simulink model "sg_pixel_blank_ML"  (Simulink 8.2)
settings: Solver=VariableStepDiscrete  StartTime=0.0  StopTime=Tsim  RelTol=1e-3
values from neighbouring files (symbols this model uses):
  ImgX = 640    [tb_pixel_blank_ML_xsvi_inout_only.m]    (also in tb_pixel_cnt.m = SizeI(2))
  ImgY = 480    [tb_pixel_blank_ML_xsvi_inout_only.m]    (also in tb_pixel_cnt.m = SizeI(1))
undefined symbols (not defined in the file or in its folder): gcbh, xlBlockLoadCallback, xlGetNormalizedPeriod
libraries: xbsIndex_r4 x73, dspsrcs4 x6
(part 1 of 2)
settings Model: Creator=sps  LastModifiedBy=tawassne
settings OptimizationCC: InitFltsAndDblsToZero=on
settings DebuggingCC: SaveWithParameterizedLinksMsg=none  SignalResolutionControl=TryResolveAllWithWarning  SolverPrmCheckMsg=none  MultiTaskDSMMsg=warning  MultiTaskCondExecSysMsg=none
settings RTWCC: IncludeERTFirstTime=on
settings GRTTargetCC: TargetFcnLib=ansi_tfl_tmw.mat

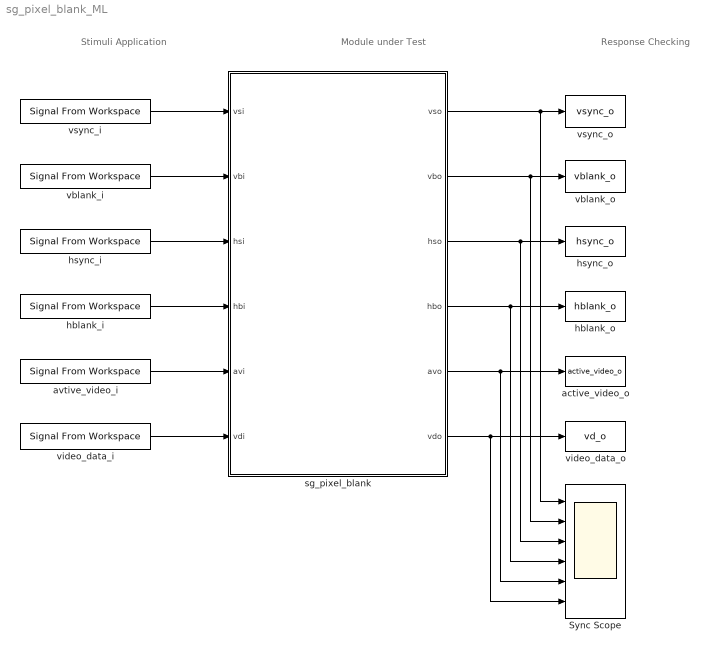
== system sg_pixel_blank_ML ==
  note: Stimuli Application
  note: Response Checking
  note: Module under Test
  Sync Scope : Scope  NumInputPorts=6
      settings: YMin=-5~-5~-5~-5~-5~-5  YMax=5~5~5~5~5~5
  active_video_o : ToWorkspace  VariableName=active_video_o  SampleTime=-1
      settings: MaxDataPoints=2*TFL
  avtive_video_i : dspsrcs4/Signal From Workspace  X=actvid_i  Ts=1  nsamps=1  OutputAfterFinalValue=Cyclic repetition  ignoreOrWarnInputAndFrameLengths=off
  hblank_i : dspsrcs4/Signal From Workspace  X=hblank_i  Ts=1  nsamps=1  OutputAfterFinalValue=Cyclic repetition  ignoreOrWarnInputAndFrameLengths=off
  hblank_o : ToWorkspace  VariableName=hblank_o  SampleTime=-1
      settings: MaxDataPoints=2*TFL
  hsync_i : dspsrcs4/Signal From Workspace  X=hsync_i  Ts=1  nsamps=1  OutputAfterFinalValue=Cyclic repetition  ignoreOrWarnInputAndFrameLengths=off
  hsync_o : ToWorkspace  VariableName=hsync_o  SampleTime=-1
      settings: MaxDataPoints=2*TFL
  sg_pixel_blank : Subsystem
  vblank_i : dspsrcs4/Signal From Workspace  X=vblank_i  Ts=1  nsamps=1  OutputAfterFinalValue=Cyclic repetition  ignoreOrWarnInputAndFrameLengths=off
  vblank_o : ToWorkspace  VariableName=vblank_o  SampleTime=-1
      settings: MaxDataPoints=2*TFL
  video_data_i : dspsrcs4/Signal From Workspace  X=vd_i  Ts=1  nsamps=1  OutputAfterFinalValue=Cyclic repetition  ignoreOrWarnInputAndFrameLengths=off
  video_data_o : ToWorkspace  VariableName=vd_o  SampleTime=-1
      settings: MaxDataPoints=2*TFL
  vsync_i : dspsrcs4/Signal From Workspace  X=vsync_i  Ts=1  nsamps=1  OutputAfterFinalValue=Cyclic repetition  ignoreOrWarnInputAndFrameLengths=off
  vsync_o : ToWorkspace  VariableName=vsync_o  SampleTime=-1
      settings: MaxDataPoints=2*TFL
  wires:
  vsync_i/1 -> sg_pixel_blank/1(vsi)
  vblank_i/1 -> sg_pixel_blank/2(vbi)
  hsync_i/1 -> sg_pixel_blank/3(hsi)
  hblank_i/1 -> sg_pixel_blank/4(hbi)
  avtive_video_i/1 -> sg_pixel_blank/5(avi)
  video_data_i/1 -> sg_pixel_blank/6(vdi)
  sg_pixel_blank/1(vso) -> vsync_o/1, Sync Scope/1
  sg_pixel_blank/2(vbo) -> vblank_o/1, Sync Scope/2
  sg_pixel_blank/3(hso) -> hsync_o/1, Sync Scope/3
  sg_pixel_blank/4(hbo) -> hblank_o/1, Sync Scope/4
  sg_pixel_blank/5(avo) -> active_video_o/1, Sync Scope/5
  sg_pixel_blank/6(vdo) -> video_data_o/1, Sync Scope/6

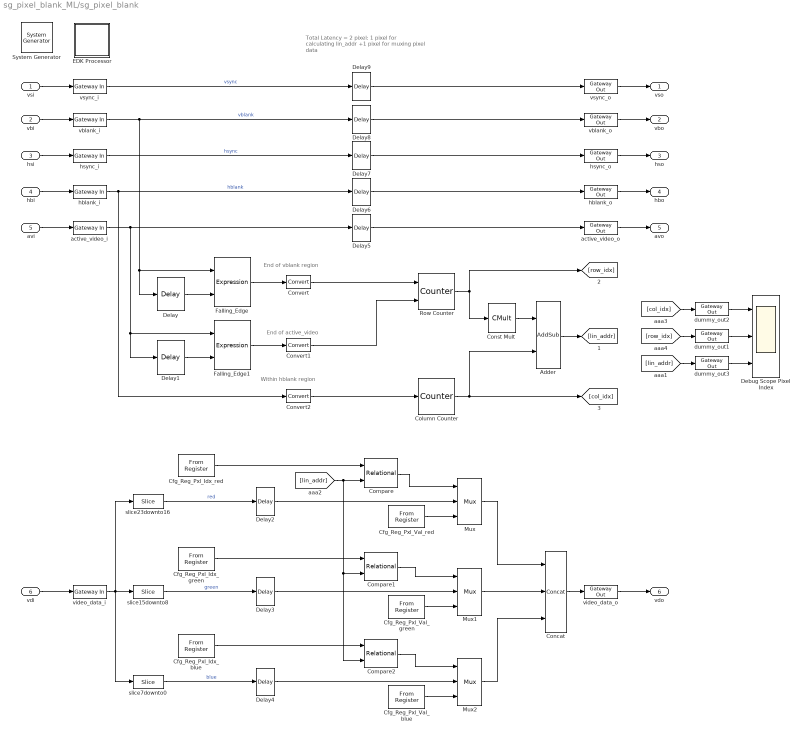
== system sg_pixel_blank_ML/sg_pixel_blank ==
  note: End of vblank region
  note: End of active_video
  note: Within hblank region
  note: Total Latency = 2 pixel:
      |     1 pixel for calculating lin_addr
      |   +1 pixel for muxing pixel data
  vsi : Inport
  vbi : Inport  Port=2
  hsi : Inport  Port=3
  hbi : Inport  Port=4
  avi : Inport  Port=5
  vdi : Inport  Port=6
  " System Generator" : xbsIndex_r4/ System Generator  Tag=genX  xilinxfamily=spartan6  part=xc6slx150t  speed=-3  package=fgg676  synthesis_tool=XST  clock_wrapper=Clock Enables  directory=./netlist  proj_type=Project Navigator  Synth_file=XST Defaults  Impl_file=ISE Defaults  testbench=off  simulink_period=1  sysclk_period=10  dcm_input_clock_period=10  incr_netlist=off  trim_vbits=Everywhere in SubSystem  dbl_ovrd=According to Block Masks  core_generation=According to Block Masks  run_coregen=off  deprecated_control=off  eval_field=0  block_type=sysgen
      settings: block_version=11.4
  Adder : xbsIndex_r4/AddSub  mode=Addition  use_carryin=off  use_carryout=off  en=off  latency=1  precision=Full  arith_type=Unsigned  n_bits=16  bin_pt=14  quantization=Truncate  overflow=Wrap  dbl_ovrd=off  use_behavioral_HDL=off  hw_selection=Fabric  pipelined=off  block_type=addsub
  Cfg_Reg_Pxl_Idx_blue : xbsIndex_r4/From Register  shared_memory_name='pixel_idx_blue'  init=70000  period=1  ownership=Locally owned and initialized  gui_display_data_type=Fixed-point  arith_type=Unsigned  n_bits=32  bin_pt=0  preci_type=Single  dbl_ovrd=off  block_type=fromreg
      settings: AttributesFormatString=<< %<shared_memory_name> >>  infoedit="Register block that reads data to a shared memory register.  Delay of one sample period."  block_version=10.1
  Cfg_Reg_Pxl_Idx_green : xbsIndex_r4/From Register  shared_memory_name='pixel_idx_green'  init=46300  period=1  ownership=Locally owned and initialized  gui_display_data_type=Fixed-point  arith_type=Unsigned  n_bits=32  bin_pt=0  preci_type=Single  dbl_ovrd=off  block_type=fromreg
      settings: AttributesFormatString=<< %<shared_memory_name> >>  infoedit="Register block that reads data to a shared memory register.  Delay of one sample period."  block_version=10.1
  Cfg_Reg_Pxl_Idx_red : xbsIndex_r4/From Register  shared_memory_name='pixel_idx_red'  init=22900  period=1  ownership=Locally owned and initialized  gui_display_data_type=Fixed-point  arith_type=Unsigned  n_bits=32  bin_pt=0  preci_type=Single  dbl_ovrd=off  block_type=fromreg
      settings: AttributesFormatString=<< %<shared_memory_name> >>  infoedit="Register block that reads data to a shared memory register.  Delay of one sample period."  block_version=10.1
  Cfg_Reg_Pxl_Val_blue : xbsIndex_r4/From Register  shared_memory_name='pixel_val_blue'  init=250  period=1  ownership=Locally owned and initialized  gui_display_data_type=Fixed-point  arith_type=Unsigned  n_bits=8  bin_pt=0  preci_type=Single  dbl_ovrd=off  block_type=fromreg
      settings: AttributesFormatString=<< %<shared_memory_name> >>  infoedit="Register block that reads data to a shared memory register.  Delay of one sample period."  block_version=10.1
  Cfg_Reg_Pxl_Val_green : xbsIndex_r4/From Register  shared_memory_name='pixel_val_green'  init=100  period=1  ownership=Locally owned and initialized  gui_display_data_type=Fixed-point  arith_type=Unsigned  n_bits=8  bin_pt=0  preci_type=Single  dbl_ovrd=off  block_type=fromreg
      settings: AttributesFormatString=<< %<shared_memory_name> >>  infoedit="Register block that reads data to a shared memory register.  Delay of one sample period."  block_version=10.1
  Cfg_Reg_Pxl_Val_red : xbsIndex_r4/From Register  shared_memory_name='pixel_val_red'  init=10  period=1  ownership=Locally owned and initialized  gui_display_data_type=Fixed-point  arith_type=Unsigned  n_bits=8  bin_pt=0  preci_type=Single  dbl_ovrd=off  block_type=fromreg
      settings: AttributesFormatString=<< %<shared_memory_name> >>  infoedit="Register block that reads data to a shared memory register.  Delay of one sample period."  block_version=10.1
  Column Counter : xbsIndex_r4/Counter  cnt_type=Count Limited  cnt_to=ImgX-1  operation=Up  start_count=0  cnt_by_val=1  arith_type=Unsigned  n_bits=ceil(log2(ImgX))  bin_pt=0  load_pin=off  rst=on  en=off  explicit_period=on  period=1  dbl_ovrd=off  use_behavioral_HDL=off  implementation=Fabric  block_type=counter
  Compare : xbsIndex_r4/Relational  mode=a<=b  en=off  latency=0  dbl_ovrd=off  block_type=relational
  Compare1 : xbsIndex_r4/Relational  mode=a<=b  en=off  latency=0  dbl_ovrd=off  block_type=relational
  Compare2 : xbsIndex_r4/Relational  mode=a<=b  en=off  latency=0  dbl_ovrd=off  block_type=relational
  Concat : xbsIndex_r4/Concat  num_inputs=3  dbl_ovrd=off  block_type=concat
  Const Mult : xbsIndex_r4/CMult  const=ImgX  gui_display_data_type=Fixed-point  const_n_bits=ceil(log2(ImgX+1))  const_bin_pt=0  float_type=Single  exp_bits=8  fraction_bits=24  en=off  latency=0  precision=Full  arith_type="Signed  (2's comp)"  n_bits=16  bin_pt=14  quantization=Truncate  overflow=Wrap  dbl_ovrd=off  use_behavioral_HDL=off  mem_type=Distributed RAM  pipeline=off  block_type=cmult
  Convert : xbsIndex_r4/Convert  gui_display_data_type=Boolean  arith_type=Boolean  n_bits=16  bin_pt=14  float_type=Single  exp_bits=8  fraction_bits=24  quantization=Truncate  overflow=Wrap  en=off  latency=0  dbl_ovrd=off  pipeline=off  block_type=convert
  Convert1 : xbsIndex_r4/Convert  gui_display_data_type=Boolean  arith_type=Boolean  n_bits=16  bin_pt=14  float_type=Single  exp_bits=8  fraction_bits=24  quantization=Truncate  overflow=Wrap  en=off  latency=0  dbl_ovrd=off  pipeline=off  block_type=convert
  Convert2 : xbsIndex_r4/Convert  gui_display_data_type=Boolean  arith_type=Boolean  n_bits=16  bin_pt=14  float_type=Single  exp_bits=8  fraction_bits=24  quantization=Truncate  overflow=Wrap  en=off  latency=0  dbl_ovrd=off  pipeline=off  block_type=convert
  Debug Scope Pixel Index : Scope  NumInputPorts=3
      settings: YMin=-5~-5~-5  YMax=5~5~5  SaveName=ScopeData2
  Delay{,1..4} (5 alike) : xbsIndex_r4/Delay  rst=off  infoeditControl=Selection of Reset will increase slice count due to use of real FFs and instead of SRLs  en=off  latency=1  dbl_ovrd=off  reg_retiming=off  block_type=delay
  Delay{5..9} (5 alike) : xbsIndex_r4/Delay  rst=off  infoeditControl=Selection of Reset will increase slice count due to use of real FFs and instead of SRLs  en=off  latency=2  dbl_ovrd=off  reg_retiming=off  block_type=delay
  EDK Processor : Subsystem  LoadFcn=xlBlockLoadCallback(gcbh);  mask(Xilinx EDK Processor Block){mode=EDK pcore generation, xmp=, MemVisToProc=<qt bgcolor="#FFFFFF"><div><img src="C:/Program_Waj/Xilinx/ISE_13.1/ISE_DS/ISE/sysgen/data/images/registerplus.gif"> &lt;&lt;pixel_idx_red&gt;&gt;<br></div><div><img src="C:/Program_Waj/Xilinx/ISE_13.1/ISE_DS/ISE/sysgen/data/images/registerplus.gif"> &lt;&lt;pixel_idx_green&gt;&gt;<br></div><div><img src="C:/Program_Waj/Xilinx/ISE_13.1/ISE_DS/ISE/sysgen/data/images/registerplus.gif"> &lt;&lt;pixel_idx_blue&gt;&gt;<br></div><div><img src="C:/Program_Waj/Xilinx/ISE_13.1/ISE_DS/ISE/sysgen/data/images/registerplus.gif"> &lt;&lt;pixel_val_red&gt;&gt;<br></div><div><img src="C:/Program_Waj/Xilinx/ISE_13.1/ISE_DS/ISE/sysgen/data/images/registerplus.gif"> &lt;&lt;pixel_val_green&gt;&gt;<br></div><div><img src="C:/Program_Waj/Xilinx/ISE_13.1/ISE_DS/ISE/sysgen/data/images/registerplus.gif"> &lt;&lt;pixel_val_blue&gt;&gt;<br></div></qt>, AvailableMemories=<empty>, portInterfaceTable={'exposed'=>[],'portdir'=>[],'portname'=>[],'shortname'=>[]}, bus_type_sgadvanced=, bus_type=PLB, baseaddr=0x80000000, baseaddr_lock_sgadvanced=, baseaddr_lock=off, dual_clock_sgadvanced=, dual_clock=on, reg_readback_sgadvanced=, reg_readback=on, ucf_file=, inheritDeviceType_sgadvanced=, inheritDeviceType=off, elf_file=, codebug_sgadvanced=, codebug=on, clock_name=plb, internalPortList={}, resetPolarity=0, memxtable={'mladdr'=>[0.00000000000000000,1.00000000000000000,2.00000000000000000,3.00000000000000000,4.00000000000000000,5.00000000000000000],'mlist'=>['sg_lens_correct_ML/sg_lens_correct/Cfg_Reg_Pxl_Idx_red','sg_lens_correct_ML/sg_lens_correct/Cfg_Reg_Pxl_Idx_green','sg_lens_correct_ML/sg_lens_correct/Cfg_Reg_Pxl_Idx_blue','sg_lens_correct_ML/sg_lens_correct/Cfg_Reg_Pxl_Val_red','sg_lens_correct_ML/sg_lens_correct/Cfg_Reg_Pxl_Val_green','sg_lens_correct_ML/sg_lens_correct/Cfg_Reg_Pxl_Val_blue'],'mlname'=>['\'pixel_idx_red\'','\'pixel_idx_green\'','\'pixel_idx_blue\'','\'pixel_val_red\'','\'pixel_val_green\'','\'pixel_val_blue\''],'mlstate'=>[0.00000000000000000,0.00000000000000000,0.00000000000000000,0.00000000000000000,0.00000000000000000,0.00000000000000000]}, procinfo={}, memmapdirty=off, blockname=, xpsintstyle=default, has_advanced_control=0, sggui_pos=-1,-1,-1,-1, block_type=edkprocessor, block_version=2.7, sg_icon_stat=55,52,-1,-1,white,blue,0,07734,right,,[ ],[ ], sg_mask_display=|, sg_list_contents={'table'=>{'AvailableMemories'=>'popup(<empty>)'}}, sg_blockgui_xml=}
      mask sg_mask_display=|
      | fprintf('','COMMENT: begin icon graphics');
      | patch([0 55 55 0 0 ],[0 0 52 52 0 ],[0.77 0.82 0.91 ]);
      | plot([0 55 55 0 0 ],[0 0 52 52 0 ]);
      | patch([11.425 21.54 28.54 35.54 42.54 28.54 18.425 11.425 ],[33.77 33.77 40.77 33.77 40.77 40.77 40.77 33.77 ],[1 1 1 ]);
      | patch([18.425 28.54 21.54 11.425 18.425 ],[26.77 26.77 33.77 33.77 26.77 ],[0.931 0.946 0.973 ]);
      | patch([11.425 21.54 28.54 18.425 11.425 ],[19.77 19.77 26.77 26.77 19.77 ],[1 1 1 ]);
      | patch([18.425 42.54 35.54 28.54 21.54 11.425 18.425 ],[12.77 12.77 19.77 12.77 19.77 19.77 12.77 ],[0.931 0.946 0.973 ]);
      | fprintf('','COMMENT: end icon graphics');
      | fprintf('','COMMENT: begin icon text');
      | fprintf('','COMMENT: end icon text');
      mask prompts: mode "Configure Processor for"; xmp "XPS Project"; MemVisToProc ""; AvailableMemories "Available Memories"; portInterfaceTable ""; bus_type_sgadvanced ""; bus_type "Bus Type"; baseaddr "Base Address"; baseaddr_lock_sgadvanced ""; baseaddr_lock "Lock"; dual_clock_sgadvanced ""; dual_clock "Dual Clocks"; reg_readback_sgadvanced ""; reg_readback "Register Read-Back"; ucf_file "Constraint File"; inheritDeviceType_sgadvanced ""; inheritDeviceType "Inherit Device Type"; elf_file "Initial Program"; codebug_sgadvanced ""; codebug "Enable Co-Debug with Xilinx SDK (Beta)"; clock_name ""; internalPortList ""; resetPolarity ""; memxtable ""; procinfo ""; memmapdirty ""; blockname ""; xpsintstyle ""; has_advanced_control ""; sggui_pos ""; block_type ""; block_version ""; sg_icon_stat ""; sg_mask_display ""; sg_list_contents ""; sg_blockgui_xml ""
      mask help: Xilinx EDK Processor
      mask init:
      | try
      |   tmp_gcb = gcb;
      |   tmp_gcbh = gcbh;
      |   if (strcmp('SysGenIndex',get_param(bdroot(tmp_gcbh),'tag')) && ~isempty(regexp(bdroot(tmp_gcb), '^xbs', 'once')))
      |     return;
      |   end;
      |   xlMungeMaskParams;
      | 
      |   block_type='edkprocessor';
      | 
      |   serialized_declarations = '{''block_type''=>''String''}';
      |   xledkprocessor_init();
      |   ptable_ = xlblockprep(get_param(tmp_gcb, 'MaskWSVariables'));
      |   try
      |     xlBlockMoveCallback(tmp_gcbh);
      |   catch 
      |      clear global xl_updateicon_recursion_guard;
      |   end;
      | catch
      |   global dbgsysgen;
      |   if(~isempty(dbgsysgen) && dbgsysgen)
      |     e = regexprep(lasterr, '\n', '\nError: ');
      |     disp(['Error: While running MaskInit code on block ' tmp_gcb ': ' e]);
      |     error(e);
      |   end
      | end
      settings: CopyFcn=xlProcBlockCopyCallback(gcbh);xlBlockMoveCallback(gcbh);  DeleteFcn=xlDestroyGui(gcbh);  ModelCloseFcn=xlDestroyGui(gcbh);  PreSaveFcn=xlBlockPreSaveCallback(gcbh);  PostSaveFcn=xlBlockPostSaveCallback(gcbh);  DestroyFcn=xlDestroyGui(gcbh);  OpenFcn=bh=gcbh;xlProcBlockCallbacks('populatesharedmemorylistbox',bh);xlOpenGui(bh, 'edkprocessor_gui.xml', @xlProcBlockEnablement, @xlProcBlockAction);  CloseFcn=xlDestroyGui(gcbh);  MoveFcn=xlBlockMoveCallback(gcbh);
      mask Help: eval('');xlDoc('-book','sysgen','-topic','EDK_Processor');
      mask TypeOptions mode: EDK pcore generation | HDL netlisting
      mask TypeOptions bus_type: AXI | PLB
      mask Display:
      | fprintf('','COMMENT: begin icon graphics');
      | patch([0 55 55 0 0 ],[0 0 52 52 0 ],[0.77 0.82 0.91 ]);
      | plot([0 55 55 0 0 ],[0 0 52 52 0 ]);
      | patch([11.425 21.54 28.54 35.54 42.54 28.54 18.425 11.425 ],[33.77 33.77 40.77 33.77 40.77 40.77 40.77 33.77 ],[1 1 1 ]);
      | patch([18.425 28.54 21.54 11.425 18.425 ],[26.77 26.77 33.77 33.77 26.77 ],[0.931 0.946 0.973 ]);
      | patch([11.425 21.54 28.54 18.425 11.425 ],[19.77 19.77 26.77 26.77 19.77 ],[1 1 1 ]);
      | patch([18.425 42.54 35.54 28.54 21.54 11.425 18.425 ],[12.77 12.77 19.77 12.77 19.77 19.77 12.77 ],[0.931 0.946 0.973 ]);
      | fprintf('','COMMENT: end icon graphics');
      | fprintf('','COMMENT: begin icon text');
      | disp('');
      | 
      | fprintf('','COMMENT: end icon text');
  Falling_Edge : xbsIndex_r4/Expression  expression=~a & b  align_bp=on  en=off  latency=0  precision=Full  arith_type=Unsigned  n_bits=16  bin_pt=0  dbl_ovrd=off  block_type=expr
  Falling_Edge1 : xbsIndex_r4/Expression  expression=~a & b  align_bp=on  en=off  latency=0  precision=Full  arith_type=Unsigned  n_bits=16  bin_pt=0  dbl_ovrd=off  block_type=expr
  Mux : xbsIndex_r4/Mux  inputs=2  en=off  latency=1  precision=Full  arith_type=Unsigned  n_bits=16  bin_pt=14  quantization=Truncate  overflow=Wrap  dbl_ovrd=off  block_type=mux
  Mux1 : xbsIndex_r4/Mux  inputs=2  en=off  latency=1  precision=Full  arith_type=Unsigned  n_bits=16  bin_pt=14  quantization=Truncate  overflow=Wrap  dbl_ovrd=off  block_type=mux
  Mux2 : xbsIndex_r4/Mux  inputs=2  en=off  latency=1  precision=Full  arith_type=Unsigned  n_bits=16  bin_pt=14  quantization=Truncate  overflow=Wrap  dbl_ovrd=off  block_type=mux
  Row Counter : xbsIndex_r4/Counter  cnt_type=Count Limited  cnt_to=ImgY-1  operation=Up  start_count=0  cnt_by_val=1  arith_type=Unsigned  n_bits=ceil(log2(ImgY))  bin_pt=0  load_pin=off  rst=on  en=on  explicit_period=on  period=1  dbl_ovrd=off  use_behavioral_HDL=off  implementation=Fabric  block_type=counter
  active_video_i : xbsIndex_r4/Gateway In  gui_display_data_type=Fixed-point  arith_type=Unsigned  n_bits=1  bin_pt=0  preci_type=Single  exp_width=8  frac_width=24  quantization="Round  (unbiased: +/- Inf)"  overflow=Saturate  period=1  dbl_ovrd=off  timing_constraint=None  locs_specified=off  LOCs={}  hdl_port=on  block_type=gatewayin
      settings: infoedit="Gateway in block.  Converts inputs of type Simulink integer, double and fixed point to  Xilinx fixed point type.<P><P>Hardware notes:  In hardware these blocks become top level input ports."  xl_area=[0, 0, 0, 0, 0, 0, 0]  block_version=VER_STRING_GOES_HERE
  active_video_o : xbsIndex_r4/Gateway Out  hdl_port=on  timing_constraint=None  locs_specified=off  LOCs={}  block_type=gatewayout
      settings: infoedit="Gateway out block.  Converts Xilinx fixed point inputs into ouputs of type Simulink integer, double, or fixed point.<P><P>Hardware notes:  In hardware these blocks become top level output ports or are discarded, depending on how they are configured."  xl_area=[0, 0, 0, 0, 0, 0, 0]  block_version=VER_STRING_GOES_HERE
  dummy_out1 : xbsIndex_r4/Gateway Out  hdl_port=off  timing_constraint=None  locs_specified=off  LOCs={}  block_type=gatewayout
      settings: infoedit="Gateway out block.  Converts Xilinx fixed point or floating-point type inputs into ouputs of type Simulink integer, double, or fixed point.<br><br>Hardware notes:  In hardware these blocks become top level output ports or are discarded, depending on how they are configured."  xl_area=[0, 0, 0, 0, 0, 0, 0]  block_version=VER_STRING_GOES_HERE
  dummy_out2 : xbsIndex_r4/Gateway Out  hdl_port=off  timing_constraint=None  locs_specified=off  LOCs={}  block_type=gatewayout
      settings: infoedit="Gateway out block.  Converts Xilinx fixed point or floating-point type inputs into ouputs of type Simulink integer, double, or fixed point.<br><br>Hardware notes:  In hardware these blocks become top level output ports or are discarded, depending on how they are configured."  xl_area=[0, 0, 0, 0, 0, 0, 0]  block_version=VER_STRING_GOES_HERE
  dummy_out3 : xbsIndex_r4/Gateway Out  hdl_port=off  timing_constraint=None  locs_specified=off  LOCs={}  block_type=gatewayout
      settings: infoedit="Gateway out block.  Converts Xilinx fixed point or floating-point type inputs into ouputs of type Simulink integer, double, or fixed point.<br><br>Hardware notes:  In hardware these blocks become top level output ports or are discarded, depending on how they are configured."  xl_area=[0, 0, 0, 0, 0, 0, 0]  block_version=VER_STRING_GOES_HERE
  hblank_i : xbsIndex_r4/Gateway In  gui_display_data_type=Fixed-point  arith_type=Unsigned  n_bits=1  bin_pt=0  preci_type=Single  exp_width=8  frac_width=24  quantization="Round  (unbiased: +/- Inf)"  overflow=Saturate  period=1  dbl_ovrd=off  timing_constraint=None  locs_specified=off  LOCs={}  hdl_port=on  block_type=gatewayin
      settings: infoedit="Gateway in block.  Converts inputs of type Simulink integer, double and fixed point to  Xilinx fixed point or floating-point data type.<br><br>Hardware notes:  In hardware these blocks become top level input ports."  xl_area=[0, 0, 0, 0, 0, 0, 0]  block_version=VER_STRING_GOES_HERE
  hblank_o : xbsIndex_r4/Gateway Out  hdl_port=on  timing_constraint=None  locs_specified=off  LOCs={}  block_type=gatewayout
      settings: infoedit="Gateway out block.  Converts Xilinx fixed point inputs into ouputs of type Simulink integer, double, or fixed point.<P><P>Hardware notes:  In hardware these blocks become top level output ports or are discarded, depending on how they are configured."  xl_area=[0, 0, 0, 0, 0, 0, 0]  block_version=VER_STRING_GOES_HERE
  hsync_i : xbsIndex_r4/Gateway In  gui_display_data_type=Fixed-point  arith_type=Unsigned  n_bits=1  bin_pt=0  preci_type=Single  exp_width=8  frac_width=24  quantization="Round  (unbiased: +/- Inf)"  overflow=Saturate  period=1  dbl_ovrd=off  timing_constraint=None  locs_specified=off  LOCs={}  hdl_port=on  block_type=gatewayin
      settings: infoedit="Gateway in block.  Converts inputs of type Simulink integer, double and fixed point to  Xilinx fixed point or floating-point data type.<br><br>Hardware notes:  In hardware these blocks become top level input ports."  xl_area=[0, 0, 0, 0, 0, 0, 0]  block_version=VER_STRING_GOES_HERE
  hsync_o : xbsIndex_r4/Gateway Out  hdl_port=on  timing_constraint=None  locs_specified=off  LOCs={}  block_type=gatewayout
      settings: infoedit="Gateway out block.  Converts Xilinx fixed point inputs into ouputs of type Simulink integer, double, or fixed point.<P><P>Hardware notes:  In hardware these blocks become top level output ports or are discarded, depending on how they are configured."  xl_area=[0, 0, 0, 0, 0, 0, 0]  block_version=VER_STRING_GOES_HERE
  slice15downto8 : xbsIndex_r4/Slice  nbits=8  boolean_output=off  mode=Lower Bit Location + Width  bit1=0  base1=MSB of Input  bit0=8  base0=LSB of Input  dbl_ovrd=off  block_type=slice
  slice23downto16 : xbsIndex_r4/Slice  nbits=8  boolean_output=off  mode=Lower Bit Location + Width  bit1=0  base1=MSB of Input  bit0=16  base0=LSB of Input  dbl_ovrd=off  block_type=slice
  slice7downto0 : xbsIndex_r4/Slice  nbits=8  boolean_output=off  mode=Lower Bit Location + Width  bit1=0  base1=MSB of Input  bit0=0  base0=LSB of Input  dbl_ovrd=off  block_type=slice
  vblank_i : xbsIndex_r4/Gateway In  gui_display_data_type=Fixed-point  arith_type=Unsigned  n_bits=1  bin_pt=0  preci_type=Single  exp_width=8  frac_width=24  quantization="Round  (unbiased: +/- Inf)"  overflow=Saturate  period=1  dbl_ovrd=off  timing_constraint=None  locs_specified=off  LOCs={}  hdl_port=on  block_type=gatewayin
      settings: infoedit="Gateway in block.  Converts inputs of type Simulink integer, double and fixed point to  Xilinx fixed point or floating-point data type.<br><br>Hardware notes:  In hardware these blocks become top level input ports."  xl_area=[0, 0, 0, 0, 0, 0, 0]  block_version=VER_STRING_GOES_HERE
  vblank_o : xbsIndex_r4/Gateway Out  hdl_port=on  timing_constraint=None  locs_specified=off  LOCs={}  block_type=gatewayout
      settings: infoedit="Gateway out block.  Converts Xilinx fixed point inputs into ouputs of type Simulink integer, double, or fixed point.<P><P>Hardware notes:  In hardware these blocks become top level output ports or are discarded, depending on how they are configured."  xl_area=[0, 0, 0, 0, 0, 0, 0]  block_version=VER_STRING_GOES_HERE
  video_data_i : xbsIndex_r4/Gateway In  gui_display_data_type=Fixed-point  arith_type=Unsigned  n_bits=24  bin_pt=0  preci_type=Single  exp_width=8  frac_width=24  quantization="Round  (unbiased: +/- Inf)"  overflow=Saturate  period=1  dbl_ovrd=off  timing_constraint=None  locs_specified=off  LOCs={}  hdl_port=on  block_type=gatewayin
      settings: infoedit="Gateway in block.  Converts inputs of type Simulink integer, double and fixed point to  Xilinx fixed point or floating-point data type.<br><br>Hardware notes:  In hardware these blocks become top level input ports."  xl_area=[0, 0, 0, 0, 0, 0, 0]  block_version=VER_STRING_GOES_HERE
  video_data_o : xbsIndex_r4/Gateway Out  hdl_port=on  timing_constraint=None  locs_specified=off  LOCs={}  block_type=gatewayout
      settings: infoedit="Gateway out block.  Converts Xilinx fixed point inputs into ouputs of type Simulink integer, double, or fixed point.<P><P>Hardware notes:  In hardware these blocks become top level output ports or are discarded, depending on how they are configured."  xl_area=[0, 0, 0, 0, 0, 0, 0]  block_version=VER_STRING_GOES_HERE
  vsync_i : xbsIndex_r4/Gateway In  gui_display_data_type=Fixed-point  arith_type=Unsigned  n_bits=1  bin_pt=0  preci_type=Single  exp_width=8  frac_width=24  quantization="Round  (unbiased: +/- Inf)"  overflow=Saturate  period=1  dbl_ovrd=off  timing_constraint=None  locs_specified=off  LOCs={}  hdl_port=on  block_type=gatewayin
      settings: infoedit="Gateway in block.  Converts inputs of type Simulink integer, double and fixed point to  Xilinx fixed point or floating-point data type.<br><br>Hardware notes:  In hardware these blocks become top level input ports."  xl_area=[0, 0, 0, 0, 0, 0, 0]  block_version=VER_STRING_GOES_HERE
  vsync_o : xbsIndex_r4/Gateway Out  hdl_port=on  timing_constraint=None  locs_specified=off  LOCs={}  block_type=gatewayout
      settings: infoedit="Gateway out block.  Converts Xilinx fixed point inputs into ouputs of type Simulink integer, double, or fixed point.<P><P>Hardware notes:  In hardware these blocks become top level output ports or are discarded, depending on how they are configured."  xl_area=[0, 0, 0, 0, 0, 0, 0]  block_version=VER_STRING_GOES_HERE
  vso : Outport
  vbo : Outport  Port=2
  hso : Outport  Port=3
  hbo : Outport  Port=4
  avo : Outport  Port=5
  vdo : Outport  Port=6
  wires:
  Row Counter/1 -> Const Mult/1, [row_idx]
  Falling_Edge/1 -> Convert/1
  dummy_out2/1 -> Debug Scope Pixel Index/1
  dummy_out1/1 -> Debug Scope Pixel Index/2
  Const Mult/1 -> Adder/1
  video_data_i/1 -> slice15downto8/1, slice23downto16/1, slice7downto0/1
  vsi/1 -> vsync_i/1
  vbi/1 -> vblank_i/1
  hsi/1 -> hsync_i/1
  hbi/1 -> hblank_i/1
  avi/1 -> active_video_i/1
  vdi/1 -> video_data_i/1
  vsync_o/1 -> vso/1
  vsync_i/1 -> Delay9/1  "vsync"
  vblank_o/1 -> vbo/1
  vblank_i/1 -> Falling_Edge/1, Delay/1, Delay8/1  "vblank"
  hsync_i/1 -> Delay7/1  "hsync"
  hsync_o/1 -> hso/1
  hblank_i/1 -> Delay6/1, Convert2/1  "hblank"
  hblank_o/1 -> hbo/1
  active_video_i/1 -> Delay1/1, Falling_Edge1/1, Delay5/1
  active_video_o/1 -> avo/1
  video_data_o/1 -> vdo/1
  Delay/1 -> Falling_Edge/2
  Delay1/1 -> Falling_Edge1/2
  Falling_Edge1/1 -> Convert1/1
  Convert/1 -> Row Counter/1
  Convert1/1 -> Row Counter/2
  Column Counter/1 -> Adder/2, [col_idx]
  Concat/1 -> video_data_o/1
  Adder/1 -> [lin_addr]
  dummy_out3/1 -> Debug Scope Pixel Index/3
  [row_idx] -> dummy_out1/1
  [col_idx] -> dummy_out2/1
  [lin_addr] -> dummy_out3/1
  [lin_addr] -> Compare/2, Compare1/2, Compare2/2
  Cfg_Reg_Pxl_Idx_red/1 -> Compare/1
  Compare/1 -> Mux/1
  slice23downto16/1 -> Delay2/1  "red"
  Cfg_Reg_Pxl_Val_red/1 -> Mux/3
  slice15downto8/1 -> Delay3/1  "green"
  Cfg_Reg_Pxl_Val_green/1 -> Mux1/3
  Cfg_Reg_Pxl_Val_blue/1 -> Mux2/3
  slice7downto0/1 -> Delay4/1  "blue"
  Mux/1 -> Concat/1
  Mux1/1 -> Concat/2
  Mux2/1 -> Concat/3
  Delay2/1 -> Mux/2
  Delay3/1 -> Mux1/2
  Delay4/1 -> Mux2/2
  Delay5/1 -> active_video_o/1
  Delay6/1 -> hblank_o/1
  Delay7/1 -> hsync_o/1
  Delay8/1 -> vblank_o/1
  Delay9/1 -> vsync_o/1
  Convert2/1 -> Column Counter/1
  Cfg_Reg_Pxl_Idx_green/1 -> Compare1/1
  Compare1/1 -> Mux1/1
  Cfg_Reg_Pxl_Idx_blue/1 -> Compare2/1
  Compare2/1 -> Mux2/1
